simulink model "FinalProject"  (R2019b)
settings: Solver=VariableStepAuto  StartTime=0.0  StopTime=10.0  RelTol=1e-3
libraries: fl_lib x24, nesl_utility x10, ee_lib x2
settings Model: Creator=dzecc  LastModifiedBy=dzecc

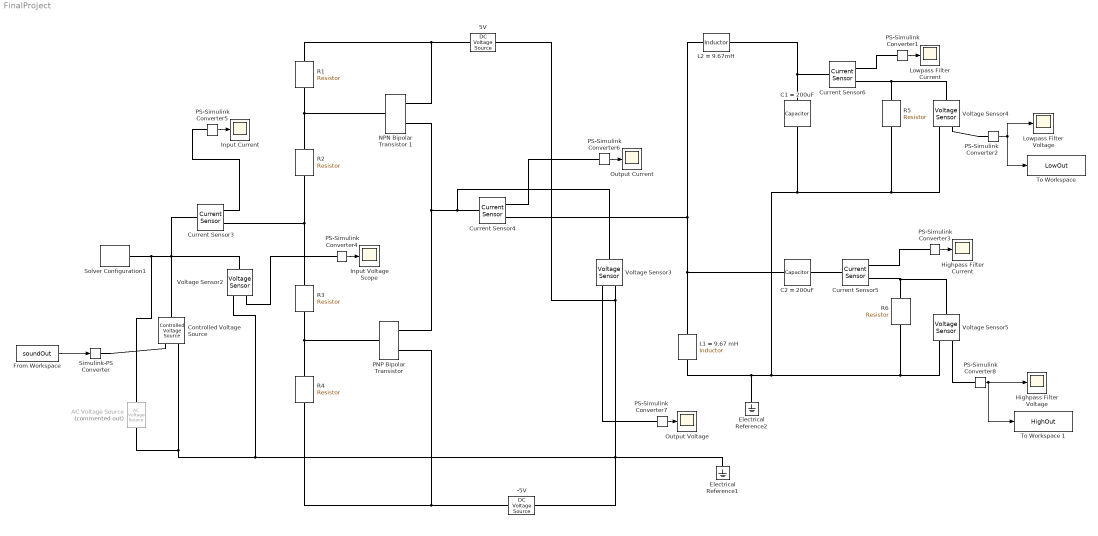
== system FinalProject ==
  -5V : fl_lib/Electrical/Electrical Sources/DC Voltage Source  v0=-5 V
  5V : fl_lib/Electrical/Electrical Sources/DC Voltage Source  v0=5 V
  "AC Voltage Source " : fl_lib/Electrical/Electrical Sources/AC Voltage Source  Commented=on  amp=1 V  shift=0 deg  frequency=80 Hz  omega=0 rad/s
  C1 = 200uF : fl_lib/Electrical/Electrical Elements/Capacitor  c=200e-6 F  r=1e-6 Ohm  g=0 1/Ohm  i_specify=off  i_priority=None  i=0 A  i_nominal_specify=off  i_nominal_unit=A  i_nominal_value=1  v_specify=off  v_priority=None  v=0 V  v_nominal_specify=off  v_nominal_unit=V  v_nominal_value=1  vc_specify=off  vc_priority=High  vc=0 V  vc_nominal_specify=off  vc_nominal_unit=V  vc_nominal_value=1
  C2 = 200uF : fl_lib/Electrical/Electrical Elements/Capacitor  c=200e-6 F  r=1e-6 Ohm  g=0 1/Ohm  i_specify=off  i_priority=None  i=0 A  i_nominal_specify=off  i_nominal_unit=A  i_nominal_value=1  v_specify=off  v_priority=None  v=0 V  v_nominal_specify=off  v_nominal_unit=V  v_nominal_value=1  vc_specify=off  vc_priority=High  vc=0 V  vc_nominal_specify=off  vc_nominal_unit=V  vc_nominal_value=1
  "Controlled Voltage Source " : fl_lib/Electrical/Electrical Sources/Controlled Voltage Source
  Current Sensor{3..6} (4 alike) : fl_lib/Electrical/Electrical Sensors/Current Sensor
  Electrical Reference1 : fl_lib/Electrical/Electrical Elements/Electrical Reference
  Electrical Reference2 : fl_lib/Electrical/Electrical Elements/Electrical Reference
  "From Workspace " : FromWorkspace  VariableName=soundOut  OutDataTypeStr=double  SampleTime=0
  Highpass Filter Current : Scope
  Highpass Filter Voltage : Scope
  Input Current : Scope
  Input Voltage Scope : Scope
  L1 = 9.67 mH : fl_lib/Electrical/Electrical Elements/Inductor  l=9.67e-3 H  r=0 Ohm  g=1e-9 1/Ohm  i_specify=off  i_priority=None  i=0 A  i_nominal_specify=off  i_nominal_unit=A  i_nominal_value=1  v_specify=off  v_priority=None  v=0 V  v_nominal_specify=off  v_nominal_unit=V  v_nominal_value=1  i_L_specify=off  i_L_priority=High  i_L=0 A  i_L_nominal_specify=off  i_L_nominal_unit=A  i_L_nominal_value=1
  L2 = 9.67mH : fl_lib/Electrical/Electrical Elements/Inductor  l=9.67e-3 H  r=0 Ohm  g=1e-9 1/Ohm  i_specify=off  i_priority=None  i=0 A  i_nominal_specify=off  i_nominal_unit=A  i_nominal_value=1  v_specify=off  v_priority=None  v=0 V  v_nominal_specify=off  v_nominal_unit=V  v_nominal_value=1  i_L_specify=off  i_L_priority=High  i_L=0 A  i_L_nominal_specify=off  i_L_nominal_unit=A  i_L_nominal_value=1
  Lowpass Filter Current : Scope
  Lowpass Filter Voltage : Scope
  NPN Bipolar Transistor 1 : ee_lib/Semiconductors & Converters/NPN Bipolar Transistor  parameterization=1  prmDatasheet=1  prmEquCoeff=1  BF=100  IS=1e-14 A  VAF=200 V  hfe=100  hoe=50e-6 1/Ohm  Ic_h=1 mA  Vce_h=5 V  V1=0.55 V  I1=0.5 mA  BR=1  Tmeas=25 degC  RC=0.01 Ohm  RE=1e-4 Ohm  RB=1 Ohm  C_BC=5 pF  C_BE=5 pF  TF=0 us  TR=0 us  hfe_T2=125  XTB=0  V1_T2=0.45 V  I1_T2=0.5 mA  Tmeas2=125 degC  EG=1.11 eV  XTI=3  ec=1  TdeviceDatasheet=25 degC  TdeviceEquCoeff=25 degC  thermal_network_parameterization=ee.enum.thermalNetworkTopology.cauer  Rth=[0, 10] K/W  Rth_Foster=[4, 6] K/W  thermal_mass_parameterization=ee.enum.thermalNetwork.timeconstant  thermal_mass=[0, 1] J/K  thermal_mass_Foster=[1.5, 3] J/K  thermal_time_constant=[0, 10] s  thermal_time_constant_Foster=[6, 18] s  thermal_mass_initial_temperatures=[25, 25] degC
      settings: SourceProductName=Simscape Electrical
  Output Current : Scope
  Output Voltage : Scope
  "PNP Bipolar Transistor " : ee_lib/Semiconductors & Converters/PNP Bipolar Transistor  parameterization=1  prmDatasheet=1  prmEquCoeff=1  BF=100  IS=1e-14 A  VAF=200 V  hfe=100  hoe=50e-6 1/Ohm  Ic_h=-1 mA  Vce_h=-5 V  V1=-0.55 V  I1=-0.5 mA  BR=1  Tmeas=25 degC  RC=0.01 Ohm  RE=1e-4 Ohm  RB=1 Ohm  C_BC=5 pF  C_BE=5 pF  TF=0 us  TR=0 us  hfe_T2=125  XTB=0  V1_T2=-0.45 V  I1_T2=-0.5 mA  Tmeas2=125 degC  EG=1.11 eV  XTI=3  ec=1  TdeviceDatasheet=25 degC  TdeviceEquCoeff=25 degC  thermal_network_parameterization=ee.enum.thermalNetworkTopology.cauer  Rth=[0, 10] K/W  Rth_Foster=[4, 6] K/W  thermal_mass_parameterization=ee.enum.thermalNetwork.timeconstant  thermal_mass=[0, 1] J/K  thermal_mass_Foster=[1.5, 3] J/K  thermal_time_constant=[0, 10] s  thermal_time_constant_Foster=[6, 18] s  thermal_mass_initial_temperatures=[25, 25] degC
      settings: SourceProductName=Simscape Electrical  SourceProductBaseCode=PS  InternalSimscapePortConfiguration="{\"Bottom\":[],\"Left\":[{\"id\":\"B\",\"label\":\"\",\"type\":\"foundation.electrical.electrical\"}],\"Right\":[{\"id\":\"n\",\"label\":\"\",\"type\":\"foundation.electrical.electrical\"},{\"id\":\"p\",\"label\":\"\",\"type\":\"foundation.electrical.electrical\"}],\"Top\":[]}"
  PS-Simulink Converter{1..8} (8 alike) : nesl_utility/PS-Simulink Converter  PhysicalDomain=network_engine_domain  SubClassName=ps_output  LeftPortType=input  RightPortType=output  PseudoPeriodic=off  Frequencies=[]  Unit=inherit  AffineConversion=off
  R1 : fl_lib/Electrical/Electrical Elements/Resistor  R=80.9 Ohm  i_specify=off  i_priority=None  i=0 A  i_nominal_specify=off  i_nominal_unit=A  i_nominal_value=1  v_specify=off  v_priority=None  v=0 V  v_nominal_specify=off  v_nominal_unit=V  v_nominal_value=1
  R2 : fl_lib/Electrical/Electrical Elements/Resistor  R=10 Ohm  i_specify=off  i_priority=None  i=0 A  i_nominal_specify=off  i_nominal_unit=A  i_nominal_value=1  v_specify=off  v_priority=None  v=0 V  v_nominal_specify=off  v_nominal_unit=V  v_nominal_value=1
  R3 : fl_lib/Electrical/Electrical Elements/Resistor  R=10 Ohm  i_specify=off  i_priority=None  i=0 A  i_nominal_specify=off  i_nominal_unit=A  i_nominal_value=1  v_specify=off  v_priority=None  v=0 V  v_nominal_specify=off  v_nominal_unit=V  v_nominal_value=1
  R4 : fl_lib/Electrical/Electrical Elements/Resistor  R=80.9 Ohm  i_specify=off  i_priority=None  i=0 A  i_nominal_specify=off  i_nominal_unit=A  i_nominal_value=1  v_specify=off  v_priority=None  v=0 V  v_nominal_specify=off  v_nominal_unit=V  v_nominal_value=1
  R5 : fl_lib/Electrical/Electrical Elements/Resistor  R=3.35 Ohm  i_specify=off  i_priority=None  i=0 A  i_nominal_specify=off  i_nominal_unit=A  i_nominal_value=1  v_specify=off  v_priority=None  v=0 V  v_nominal_specify=off  v_nominal_unit=V  v_nominal_value=1
  R6 : fl_lib/Electrical/Electrical Elements/Resistor  R=4 Ohm  i_specify=off  i_priority=None  i=0 A  i_nominal_specify=off  i_nominal_unit=A  i_nominal_value=1  v_specify=off  v_priority=None  v=0 V  v_nominal_specify=off  v_nominal_unit=V  v_nominal_value=1
  "Simulink-PS Converter " : nesl_utility/Simulink-PS Converter  PhysicalDomain=network_engine_domain  SubClassName=ps_input  LeftPortType=input  RightPortType=output  PseudoPeriodic=off  Frequencies=[]  NoiseDistribution=none  NoiseParameters=[]  Unit=1  AffineConversion=off  FilteringAndDerivatives=provide  SimscapeFilterOrder=1  InputFilterTimeConstant=0.001  UdotUserProvided=0
  "Solver Configuration1 " : nesl_utility/Solver Configuration  PhysicalDomain=network_engine_domain  SubClassName=solver  LeftPortType=input  RightPortType=generic  Tones=[]  Harmonics=[]  SimulateNoise=off  Profile=off  UseLocalSampling=off  EnableSwitchedLinearOptims=on  FrequencyDomain=off  UseCCode=off  RelTol=0.001  AbsTol=1e-06  MinStep=1e-09  ToWorkspace=off  RevertToSquareIcSolve=off  NumHomotopyIterations=100  PhasorMode=off  PhasorModeNumHarmonics=1  DoDC=off  ResidualTolerance=1e-09  UseLocalSolver=off  LocalSolverChoice=NE_BACKWARD_EULER_ADVANCER  LocalSolverSampleTime=0.001  DoFixedCost=off  MaxNonlinIter=3  MaxModeIter=2  LinearAlgebra=auto  EquationFormulation=NE_TIME_EF  DelaysMemoryBudget=1024  AutomaticFiltering=on  FilteringTimeConstant=0.001  PartitionStorageMethod=AS_NEEDED  PartitionMemoryBudget=1024  PartitionMethod=ROBUST
  "To Workspace " : ToWorkspace  VariableName=LowOut  SampleTime=-1
  To Workspace 1 : ToWorkspace  VariableName=HighOut  SampleTime=-1
  Voltage Sensor{2..5} (4 alike) : fl_lib/Electrical/Electrical Sensors/Voltage Sensor
  wires:
  "From Workspace "/1 -> "Simulink-PS Converter "/1
  PS-Simulink Converter4/1 -> Input Voltage Scope/1
  PS-Simulink Converter5/1 -> Input Current/1
  PS-Simulink Converter6/1 -> Output Current/1
  PS-Simulink Converter7/1 -> Output Voltage/1
  PS-Simulink Converter1/1 -> Lowpass Filter Current/1
  PS-Simulink Converter2/1 -> "To Workspace "/1, Lowpass Filter Voltage/1
  PS-Simulink Converter3/1 -> Highpass Filter Current/1
  PS-Simulink Converter8/1 -> To Workspace 1/1, Highpass Filter Voltage/1
  connections:
  "Controlled Voltage Source "/LConn1 -- "AC Voltage Source "/LConn1 -- "Solver Configuration1 "/RConn1 -- Voltage Sensor2/LConn1 -- Current Sensor3/LConn1
  "Simulink-PS Converter "/RConn1 -- "Controlled Voltage Source "/RConn1
  R2/LConn1 -- NPN Bipolar Transistor 1/LConn1 -- R1/RConn1
  R2/RConn1 -- Current Sensor3/RConn2 -- R3/LConn1
  R3/RConn1 -- R4/LConn1 -- "PNP Bipolar Transistor "/LConn1
  Electrical Reference1/LConn1 -- 5V/RConn1 -- Voltage Sensor3/RConn2 -- -5V/RConn1 -- Voltage Sensor2/RConn2 -- "AC Voltage Source "/RConn1 -- "Controlled Voltage Source "/RConn2
  NPN Bipolar Transistor 1/RConn2 -- Voltage Sensor3/LConn1 -- Current Sensor4/LConn1 -- "PNP Bipolar Transistor "/RConn1
  R1/LConn1 -- NPN Bipolar Transistor 1/RConn1 -- 5V/LConn1
  R4/RConn1 -- "PNP Bipolar Transistor "/RConn2 -- -5V/LConn1
  L2 = 9.67mH/LConn1 -- Current Sensor4/RConn2 -- C2 = 200uF/LConn1 -- L1 = 9.67 mH/LConn1
  Current Sensor5/LConn1 -- C2 = 200uF/RConn1
  C1 = 200uF/LConn1 -- Current Sensor6/LConn1 -- L2 = 9.67mH/RConn1
  Current Sensor6/RConn2 -- Voltage Sensor4/LConn1 -- R5/LConn1
  Current Sensor5/RConn2 -- Voltage Sensor5/LConn1 -- R6/LConn1
  L1 = 9.67 mH/RConn1 -- Electrical Reference2/LConn1 -- R5/RConn1 -- Voltage Sensor4/RConn2 -- C1 = 200uF/RConn1 -- R6/RConn1 -- Voltage Sensor5/RConn2
  Voltage Sensor2/RConn1 -- PS-Simulink Converter4/LConn1
  Current Sensor3/RConn1 -- PS-Simulink Converter5/LConn1
  Current Sensor4/RConn1 -- PS-Simulink Converter6/LConn1
  Voltage Sensor3/RConn1 -- PS-Simulink Converter7/LConn1
  PS-Simulink Converter1/LConn1 -- Current Sensor6/RConn1
  PS-Simulink Converter2/LConn1 -- Voltage Sensor4/RConn1
  Current Sensor5/RConn1 -- PS-Simulink Converter3/LConn1
  Voltage Sensor5/RConn1 -- PS-Simulink Converter8/LConn1
